simulink model "Cruise"  (R2019b)
settings: Solver=VariableStepAuto  StartTime=0.0  StopTime=10  RelTol=1e-3
values from neighbouring files (symbols this model uses):
  b = 50    [cruiseParam.m]
  Ki = 40    [cruiseParam.m]
  Kp = 800    [cruiseParam.m]
  m = 1000    [cruiseParam.m]
  r = 10    [cruiseParam.m]
settings Model: Creator=zhaoyuan_huo  LastModifiedBy=zhaoyuan_huo

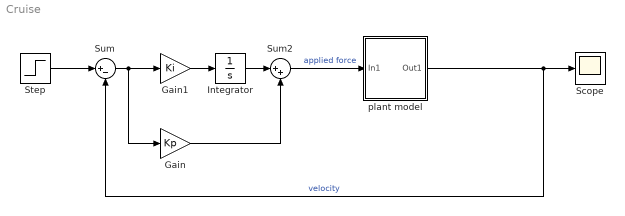
== system Cruise ==
  Gain : Gain  Gain=Kp
  Gain1 : Gain  Gain=Ki
  Integrator : Integrator
  Scope : Scope
  Step : Step  Time=0  After=r  SampleTime=0
  Sum : Sum  Inputs=|+-
  Sum2 : Sum  Inputs=|++
  plant model : Subsystem
  wires:
  plant model/1(Out1) -> Scope/1, Sum/2  "velocity"
  Sum/1 -> Gain1/1, Gain/1
  Step/1 -> Sum/1
  Gain1/1 -> Integrator/1
  Integrator/1 -> Sum2/1
  Gain/1 -> Sum2/2
  Sum2/1 -> plant model/1(In1)  "applied force"

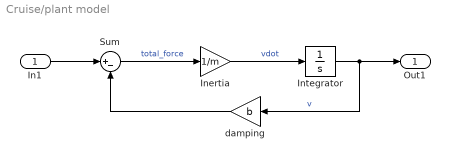
== system Cruise/plant model ==
  In1 : Inport
  Inertia : Gain  Gain=1/m
  Integrator : Integrator
  Sum : Sum  Inputs=|+-
  damping : Gain  Gain=b
  Out1 : Outport
  wires:
  Inertia/1 -> Integrator/1  "vdot"
  Sum/1 -> Inertia/1  "total_force"
  damping/1 -> Sum/2
  Integrator/1 -> Out1/1, damping/1  "v"
  In1/1 -> Sum/1
